simulink model "ADRC"  (R2022b)
settings: Solver=VariableStepAuto  StartTime=0.0  StopTime=10.0  RelTol=1e-3
values from neighbouring files (symbols this model uses):
  ModelParam_I_xx = 0.0211    [MPC.m]    (also in Quadrotor_parameters.m)
  ModelParam_I_yy = 0.0219    [MPC.m]    (also in Quadrotor_parameters.m)
  ModelParam_I_zz = 0.0366    [MPC.m]    (also in Quadrotor_parameters.m)
settings Model: Creator=12854  LastModifiedBy=12854

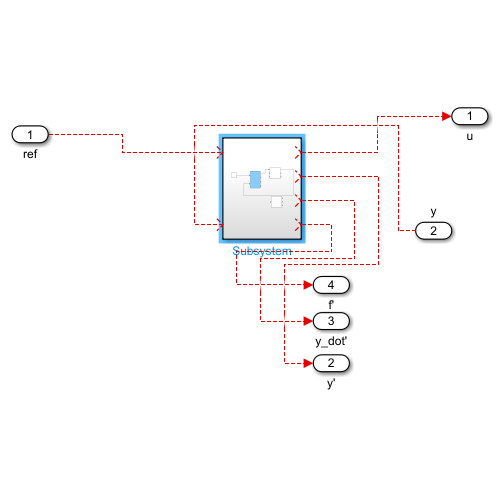
[thumbnail: Simulink's stored preview of the top-level diagram]
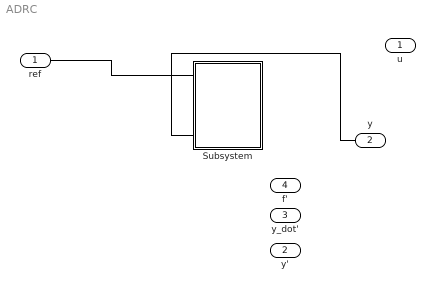
== system ADRC ==
  ref : Inport
  y : Inport  Port=2
  Subsystem : Subsystem
  u : Outport  VectorParamsAs1DForOutWhenUnconnected=off
  y' : Outport  Port=2  VectorParamsAs1DForOutWhenUnconnected=off
  y_dot' : Outport  Port=3  VectorParamsAs1DForOutWhenUnconnected=off
  f' : Outport  Port=4  VectorParamsAs1DForOutWhenUnconnected=off
  wires:
  ref/1 -> ?
  y/1 -> ?
  ? -> u/1
  ? -> y'/1
  ? -> y_dot'/1
  ? -> f'/1

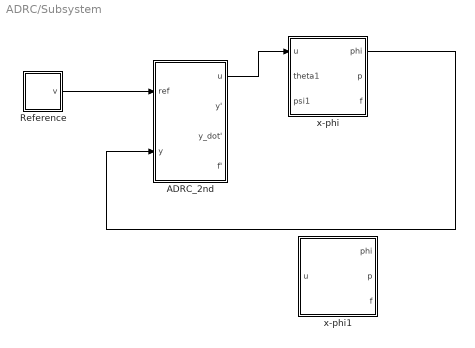
== system ADRC/Subsystem ==
  ADRC_2nd : Subsystem
  Reference : Subsystem
  x-phi : Subsystem
  x-phi1 : Subsystem
  wires:
  ADRC_2nd/1(u) -> x-phi/1(u)
  x-phi/1(phi) -> ADRC_2nd/2(y)
  Reference/1(v) -> ADRC_2nd/1(ref)

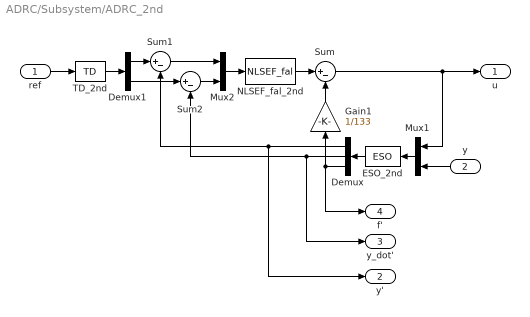
== system ADRC/Subsystem/ADRC_2nd ==
  ref : Inport
  y : Inport  Port=2
  Demux : Demux  Outputs=3
  Demux1 : Demux  Outputs=2
  ESO_2nd : S-Function  FunctionName=ESO  Parameters=CtrlPara  SFunctionDeploymentMode=off  EnableBusSupport=off
  Gain1 : Gain  Gain=1/133
  Mux1 : Mux  Inputs=2
  Mux2 : Mux  Inputs=2
  NLSEF_fal_2nd : S-Function  FunctionName=NLSEF_fal  Parameters=CtrlPara  SFunctionDeploymentMode=off  EnableBusSupport=off
  Sum : Sum  Inputs=|+-
  Sum1 : Sum  Inputs=|+-
  Sum2 : Sum  Inputs=|+-
  TD_2nd : S-Function  FunctionName=TD  Parameters=CtrlPara  SFunctionDeploymentMode=off  EnableBusSupport=off
  u : Outport  VectorParamsAs1DForOutWhenUnconnected=off
  y' : Outport  Port=2  VectorParamsAs1DForOutWhenUnconnected=off
  y_dot' : Outport  Port=3  VectorParamsAs1DForOutWhenUnconnected=off
  f' : Outport  Port=4  VectorParamsAs1DForOutWhenUnconnected=off
  wires:
  Mux2/1 -> NLSEF_fal_2nd/1
  ESO_2nd/1 -> Demux/1
  Demux1/2 -> Sum2/1
  ref/1 -> TD_2nd/1
  Demux/1 -> y'/1, Sum1/2
  TD_2nd/1 -> Demux1/1
  y/1 -> Mux1/2
  Gain1/1 -> Sum/2
  Demux/2 -> y_dot'/1, Sum2/2
  Demux1/1 -> Sum1/1
  Demux/3 -> Gain1/1, f'/1
  Sum2/1 -> Mux2/2
  Sum/1 -> Mux1/1, u/1
  NLSEF_fal_2nd/1 -> Sum/1
  Sum1/1 -> Mux2/1
  Mux1/1 -> ESO_2nd/1

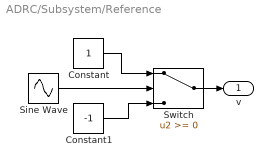
== system ADRC/Subsystem/Reference ==
  Constant : Constant
  Constant1 : Constant  Value=-1
  Sine Wave : Sin  Frequency=0.75  SampleTime=0
  Switch : Switch  SaturateOnIntegerOverflow=off  InputSameDT=off
  v : Outport  VectorParamsAs1DForOutWhenUnconnected=off
  wires:
  Constant1/1 -> Switch/3
  Sine Wave/1 -> Switch/2
  Constant/1 -> Switch/1
  Switch/1 -> v/1

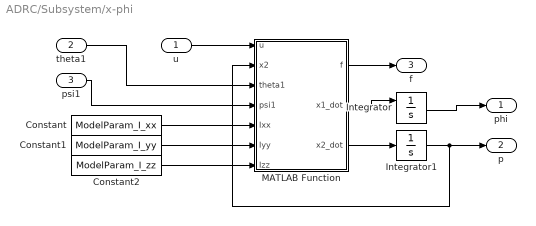
== system ADRC/Subsystem/x-phi ==
  u : Inport
  theta1 : Inport  Port=2
  psi1 : Inport  Port=3
  Constant : Constant  Value=ModelParam_I_xx
  Constant1 : Constant  Value=ModelParam_I_yy
  Constant2 : Constant  Value=ModelParam_I_zz
  Integrator : Integrator  InitialConditionSource=external
  Integrator1 : Integrator
  MATLAB Function : MATLAB Function  TreatAsAtomicUnit=on
  phi : Outport  VectorParamsAs1DForOutWhenUnconnected=off
  p : Outport  Port=2  VectorParamsAs1DForOutWhenUnconnected=off
  f : Outport  Port=3  VectorParamsAs1DForOutWhenUnconnected=off
  wires:
  u/1 -> MATLAB Function/1(u)
  MATLAB Function/2(x1_dot) -> Integrator/1
  MATLAB Function/1(f) -> f/1
  Integrator1/1 -> MATLAB Function/2(x2), p/1
  MATLAB Function/3(x2_dot) -> Integrator1/1
  Integrator/1 -> phi/1
  Constant/1 -> MATLAB Function/5(Ixx)
  Constant1/1 -> MATLAB Function/6(Iyy)
  Constant2/1 -> MATLAB Function/7(Izz)
  theta1/1 -> MATLAB Function/3(theta1)
  psi1/1 -> MATLAB Function/4(psi1)

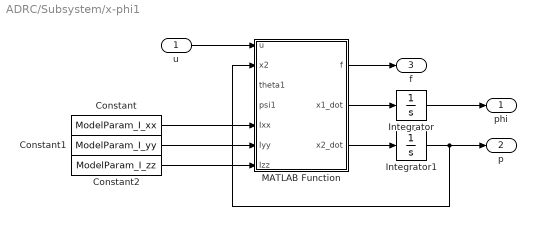
== system ADRC/Subsystem/x-phi1 ==
  u : Inport
  Constant : Constant  Value=ModelParam_I_xx
  Constant1 : Constant  Value=ModelParam_I_yy
  Constant2 : Constant  Value=ModelParam_I_zz
  Integrator : Integrator
  Integrator1 : Integrator
  MATLAB Function : MATLAB Function  TreatAsAtomicUnit=on
  phi : Outport  VectorParamsAs1DForOutWhenUnconnected=off
  p : Outport  Port=2  VectorParamsAs1DForOutWhenUnconnected=off
  f : Outport  Port=3  VectorParamsAs1DForOutWhenUnconnected=off
  wires:
  u/1 -> MATLAB Function/1(u)
  MATLAB Function/2(x1_dot) -> Integrator/1
  MATLAB Function/1(f) -> f/1
  Integrator1/1 -> MATLAB Function/2(x2), p/1
  MATLAB Function/3(x2_dot) -> Integrator1/1
  Integrator/1 -> phi/1
  Constant/1 -> MATLAB Function/5(Ixx)
  Constant1/1 -> MATLAB Function/6(Iyy)
  Constant2/1 -> MATLAB Function/7(Izz)

== matlab function ADRC/Subsystem/x-phi1/MATLAB Function ==
  data: u input; x2 input; f output; theta1 input; x1_dot output; x2_dot output; psi1 input; Ixx input; Iyy input; Izz input
function [f, x1_dot, x2_dot] = fcn(u, x2, theta1, psi1, Ixx, Iyy, Izz)

x1_dot = x2;
x2_dot = (Iyy-Izz)/Txx*theta1*psi1+u/Ixx;
f = (Iyy-Izz)/Txx*theta1*psi1;
end

== matlab function ADRC/Subsystem/x-phi/MATLAB Function ==
  data: u input; x2 input; f output; theta1 input; x1_dot output; x2_dot output; psi1 input; Ixx input; Iyy input; Izz input
function [f, x1_dot, x2_dot] = fcn(u, x2, theta1, psi1, Ixx, Iyy, Izz)

x1_dot = x2;
x2_dot = (Iyy-Izz)/Txx*theta1*psi1+u/Ixx;
f = (Iyy-Izz)/Txx*theta1*psi1;
end
